simulink model "UnderstandingBodePlot"  (R2021a)
settings: Solver=VariableStepAuto  StartTime=0.0  StopTime=30  RelTol=1e-3
settings Model: Creator=Hyukjun Kwon  LastModifiedBy=Hyukjun Kwon

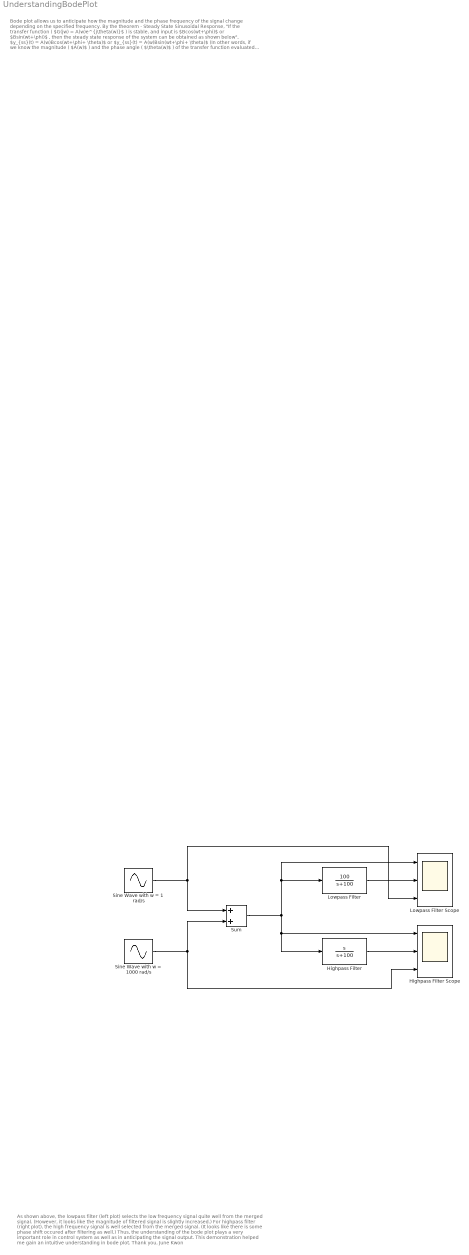
== system UnderstandingBodePlot ==
  note: As shown above, the lowpass filter (left plot) selects the low frequency signal quite well from the merged signal.
      | (However, it looks like the magnitude of filtered signal is slightly increased.)
      |
      | For highpass filter (right plot), the high frequency signal is well selected from the merged signal.
      | (It looks like there is some phase shift occured after filtering as well.)
      |
      | Thus, the understanding of the bode plot plays a very important role in control system as well as in anticipating the signal output. This demonstration helped me gain an intuitive understanding in bode plot.
      |
      | Thank you,
      | June Kwon
  note: Bode plot allows us to anticipate how the magnitude and the phase frequency of the signal change depending on the specified frequency.
      |
      | By the theorem - Steady State Sinusoidal Response, "If the transfer function ( $G(jw) = A(w)e^{j\theta(w)}$ ) is stable, and input is $Bcos(wt+\phi)$ or $Bsin(wt+\phi)$ , then the steady state response of the system can be obtained as shown below",
      |
      | $y_{ss}(t) = A(w)Bcos(wt+\phi+ \theta)$ or $y_{ss}(t) = A(w)Bsin(wt+\phi+ \theta)$
      |
      | (In other words, if we know the magnitude ( $A(w)$ ) and the phase angle ( $\theta(w)$ ) of the transfer function evaluated at a specific frequency, $w$ , and we know the magnitude ( $B$ ) and the phase angle ( $\phi$ ) of the input signal, then we can obtain the steady state response of the system by using above equation.)
      |
      | Moreover, given the system, the bode plot can be drawn by the linear combination of the magnitude and phase frequency response of zeros and poles of the transfer function. (In other words, the bode plot of the "whole" system can be drived by linear combination (summation) of each bode plot of zeros and poles of the transfer function.)
      |
      | Thus, once properly understanding the bode plot, one can then design a lowpass or a highpass filter to selectively reject signals in certain frequency ranges.
      |
      | For example, a lowpass filter and a highpass filter can be designed as shown below.
      |
      | Lowpass: $\frac{100}{s+100}$ , Highpass: $\frac{s}{s+100}$
      | whose bode plots look like...
      |
      | where the left plot represents the bode plot of the lowpass filter, and right represents the highpass filter.
      |
      | As shown above, the bode plot of the lowpass filter implies that the signal with less than 100 rad/s frequency (cut-off frequency) will have no change in magnitude (= 0 dB = 1), but the signal with higher than 100 rad/s frequency will have a decreased magnitude (= -# dB).
      |
      | Also, the bode plot of the highpass filter implies that the signal with less than 100 rad/s frequency will have decreased magnitude (= -# dB), and the signal with higher than 100 rad/s frequency will have the same magnitude as the input signal (= 0 dB = 1).
      |
      | (Please note: For passed signals, the magnitude will not exactly be the same. It will be very close to the same. Also, even if the signal passed the filter, there could be slight change in the phase angle as well...!)
      |
      | Thus, for demonstration, a simulink model for both the lowpass filter and the highpass filter have been made.
      | Two sine wave signals, one with w = 1 rad/s and the other with w = 1000 rad/s, will be merged and go through the lowpass filter and the highpass filter.
      |
      | Since the cut-off frequency of both filters are 100 rad/s, it is my expectation that, from the merged signal, for lowpass filter, the signal with low frequency (w = 1 rad/s) will be selected, and the high frequency (w = 1000 rad/s) will be rejected. For highpass fitler, the high frequency signal will be selected, and the low frequency will be rejected.
      |
      | Below is the result.
  Highpass Filter : TransferFcn  Numerator=[1 0]  Denominator=[1 100]
  Highpass Filter Scope : Scope  NumInputPorts=3
  Lowpass Filter : TransferFcn  Numerator=[100]  Denominator=[1 100]
  Lowpass Filter Scope : Scope  NumInputPorts=3
  Sine Wave with w = 1 rad/s : Sin  SampleTime=0
  Sine Wave with w = 1000 rad/s : Sin  Frequency=1000  SampleTime=0
  Sum : Sum
  wires:
  Sine Wave with w = 1000 rad/s/1 -> Sum/2, Highpass Filter Scope/3
  Sine Wave with w = 1 rad/s/1 -> Sum/1, Lowpass Filter Scope/3
  Sum/1 -> Lowpass Filter Scope/1, Lowpass Filter/1, Highpass Filter/1, Highpass Filter Scope/1
  Lowpass Filter/1 -> Lowpass Filter Scope/2
  Highpass Filter/1 -> Highpass Filter Scope/2
